simulink model "Contol_PID_OPC_Tanque02"  (R2013a)
settings: Solver=ode45  StartTime=0.0  StopTime=400  RelTol=1e-3
PreLoadFcn:
  | load('Kp.mat')
  | load('Kd.mat')
  | load('Ki.mat')
  | load('Kpm.mat')
  | load('Kdm.mat')
  | load('Kim.mat')
InitFcn:
  | load('Kp.mat')
  | load('Kd.mat')
  | load('Ki.mat')
  | load('Kpm.mat')
  | load('Kdm.mat')
  | load('Kim.mat')
values from neighbouring files (symbols this model uses):
  Kd = -2.1308168557    [Kd.mat]
  Kdm = x(3)    [Funcion_Objetivo_PID.m]    (also in Kdm.mat = 1.60825262821)
  Ki = 0.22046236166    [Kd.mat]
  Kim = x(2)    [Funcion_Objetivo_PID.m]    (also in Kdm.mat = -0.37973848981)
  Kp = 4.86450734815    [Kd.mat]
  Kpm = x(1)    [Funcion_Objetivo_PID.m]    (also in Kdm.mat = 0.790500863568)
undefined symbols (not defined in the file or in its folder): sigbuilder_block
libraries: opclib x4, simulink x2
settings Model: Creator=alvares  LastModifiedBy=alvares

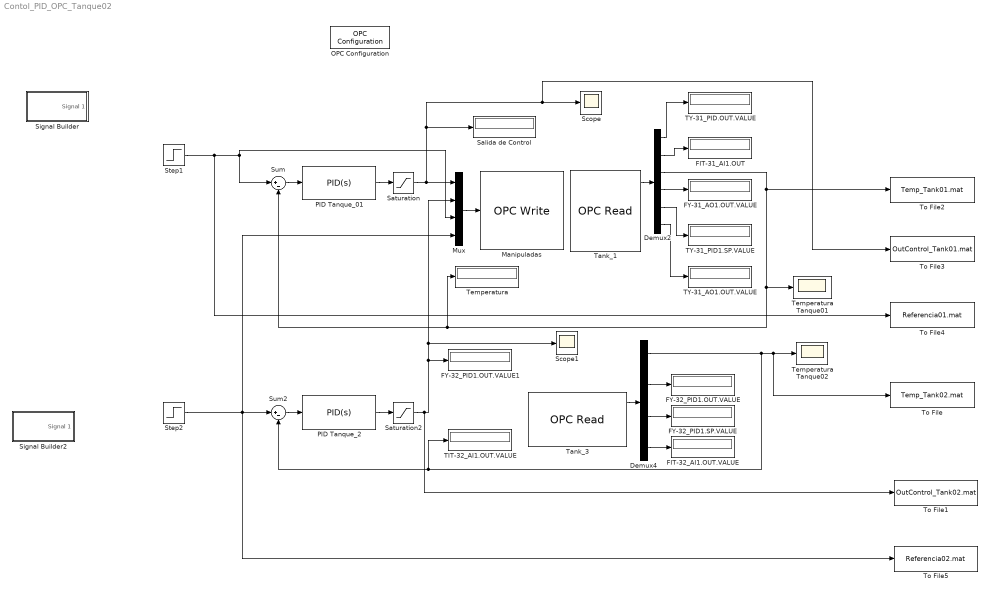
== system Contol_PID_OPC_Tanque02 ==
  Demux2 : Demux  Outputs=6
  Demux4 : Demux
  FIT-31_AI1.OUT : Display
  FIT-32_AI1.OUT.VALUE : Display
  FY-31_AO1.OUT.VALUE : Display
  FY-32_PID1.OUT.VALUE : Display
  FY-32_PID1.OUT.VALUE1 : Display
  FY-32_PID1.SP.VALUE : Display
  Manipuladas : opclib/OPC Write  serverHost=164.41.17.129  serverID=Smar.DfiOleServer.0  itemIDs=TY-31_PID1.OUT.VALUE, FY-32_PID1.OUT.VALUE, TY-31_PID1.SP.VALUE, FY-32_PID1.SP.VALUE  writeMode=Synchronous  updateRate=0.5
  Mux : Mux
  OPC Configuration : opclib/OPC Configuration  opcServers=164.41.17.129/Smar.DfiOleServer.0/10  errMissingItems=Error  errReadWrite=Warn  errShutdown=Error  errRTViolation=Warn  rtEnable=on  speedup=1  showLatency=off  beingUsed=on
  PID Tanque_01 : simulink/Continuous/PID Controller  Controller=PID  TimeDomain=Continuous-time  SampleTime=1  IntegratorMethod=Forward Euler  FilterMethod=Forward Euler  Form=Parallel  P=Kp  I=Ki  D=Kd  N=100  InitialConditionSource=internal  InitialConditionForIntegrator=0  InitialConditionForFilter=0  ExternalReset=none  ZeroCross=off  LimitOutput=off  UpperSaturationLimit=inf  LowerSaturationLimit=-inf  LinearizeAsGain=on  AntiWindupMode=none  Kb=1  TrackingMode=off  Kt=1  PParamMin=[]  PParamMax=[]  IParamMin=[]  IParamMax=[]  DParamMin=[]  DParamMax=[]  NParamMin=[]  NParamMax=[]  KbParamMin=[]  KbParamMax=[]  KtParamMin=[]  KtParamMax=[]  POutMin=[]  POutMax=[]  IOutMin=[]  IOutMax=[]  DOutMin=[]  DOutMax=[]  NOutMin=[]  NOutMax=[]  KbOutMin=[]  KbOutMax=[]  KtOutMin=[]  KtOutMax=[]  IntegratorOutMin=[]  IntegratorOutMax=[]  FilterOutMin=[]  FilterOutMax=[]  SumOutMin=[]  SumOutMax=[]  SumI1OutMin=[]  SumI1OutMax=[]  SumI2OutMin=[]  SumI2OutMax=[]  SumI3OutMin=[]  SumI3OutMax=[]  SumDOutMin=[]  SumDOutMax=[]  SaturationOutMin=[]  SaturationOutMax=[]  IntegratorContinuousStateAttributes=''  IntegratorStateMustResolveToSignalObject=off  IntegratorRTWStateStorageClass=Auto  FilterContinuousStateAttributes=''  FilterStateMustResolveToSignalObject=off  FilterRTWStateStorageClass=Auto
  PID Tanque_2 : simulink/Continuous/PID Controller  Controller=PID  TimeDomain=Continuous-time  SampleTime=1  IntegratorMethod=Forward Euler  FilterMethod=Forward Euler  Form=Parallel  P=Kpm  I=Kim  D=Kdm  N=100  InitialConditionSource=internal  InitialConditionForIntegrator=0  InitialConditionForFilter=0  ExternalReset=none  LimitOutput=off  UpperSaturationLimit=inf  LowerSaturationLimit=-inf  LinearizeAsGain=on  AntiWindupMode=none  Kb=1  TrackingMode=off  Kt=1  PParamMin=[]  PParamMax=[]  IParamMin=[]  IParamMax=[]  DParamMin=[]  DParamMax=[]  NParamMin=[]  NParamMax=[]  KbParamMin=[]  KbParamMax=[]  KtParamMin=[]  KtParamMax=[]  POutMin=[]  POutMax=[]  IOutMin=[]  IOutMax=[]  DOutMin=[]  DOutMax=[]  NOutMin=[]  NOutMax=[]  KbOutMin=[]  KbOutMax=[]  KtOutMin=[]  KtOutMax=[]  IntegratorOutMin=[]  IntegratorOutMax=[]  FilterOutMin=[]  FilterOutMax=[]  SumOutMin=[]  SumOutMax=[]  SumI1OutMin=[]  SumI1OutMax=[]  SumI2OutMin=[]  SumI2OutMax=[]  SumI3OutMin=[]  SumI3OutMax=[]  SumDOutMin=[]  SumDOutMax=[]  SaturationOutMin=[]  SaturationOutMax=[]  IntegratorContinuousStateAttributes=''  IntegratorStateMustResolveToSignalObject=off  IntegratorRTWStateStorageClass=Auto  FilterContinuousStateAttributes=''  FilterStateMustResolveToSignalObject=off  FilterRTWStateStorageClass=Auto
  Salida de Control : Display
  Saturation : Saturate  UpperLimit=100  LowerLimit=-100  ZeroCross=off
  Saturation2 : Saturate  UpperLimit=100  LowerLimit=-100  ZeroCross=off
  Scope : Scope
      settings: SaveName=Saida_PID_AQUECIMENTO
  Scope1 : Scope
      settings: SaveName=Saida_PID_MISTURA
  Signal Builder : Subsystem  Tag=STV Subsys  LoadFcn=sigbuilder_block('load');  StartFcn=sigbuilder_block('start');  StopFcn=sigbuilder_block('stop');  ClipboardFcn=sigbuilder_block('clipboard');  mask(Sigbuilder block){}
      mask help: Simulink:masks:SigbuilderBlock_MD
      mask init:
      | if ~strcmp(get_param(bdroot(gcbh),'SimulationStatus'),'stopped') tuvar = sigbuilder_block('maskInit'); end
      settings: CopyFcn=sigbuilder_block('copy');  DeleteFcn=sigbuilder_block('delete');  ModelCloseFcn=sigbuilder_block('modelClose');  PreSaveFcn=sigbuilder_block('preSave');  PauseFcn=sigbuilder_block('pause');  ContinueFcn=sigbuilder_block('continue');  NameChangeFcn=sigbuilder_block('namechange');  OpenFcn=sigbuilder_block('open',[6 28.5 1012.5 484.5 ]);  CloseFcn=sigbuilder_block('close');
      mask Display: plot(0, 0, 100, 100,[2, 2, 32, 32, 2], [68, 8, 8, 68, 68],[32, 2], [38, 38], [32, 19, 2],[53, 60, 44], [32, 17, 17, 2],[16, 16, 31, 31]);txt = getActiveGroup(gcbh);text(2, 100, txt,'verticalAlignment', 'top');
  Signal Builder2 : Subsystem  Tag=STV Subsys  LoadFcn=sigbuilder_block('load');  StartFcn=sigbuilder_block('start');  StopFcn=sigbuilder_block('stop');  ClipboardFcn=sigbuilder_block('clipboard');  mask(Sigbuilder block){}
      mask help: Simulink:masks:SigbuilderBlock_MD
      mask init:
      | if ~strcmp(get_param(bdroot(gcbh),'SimulationStatus'),'stopped') tuvar = sigbuilder_block('maskInit'); end
      settings: CopyFcn=sigbuilder_block('copy');  DeleteFcn=sigbuilder_block('delete');  ModelCloseFcn=sigbuilder_block('modelClose');  PreSaveFcn=sigbuilder_block('preSave');  PauseFcn=sigbuilder_block('pause');  ContinueFcn=sigbuilder_block('continue');  NameChangeFcn=sigbuilder_block('namechange');  OpenFcn=sigbuilder_block('open',[6 28.5 1012.5 484.5 ]);  CloseFcn=sigbuilder_block('close');
      mask Display: plot(0, 0, 100, 100,[2, 2, 32, 32, 2], [68, 8, 8, 68, 68],[32, 2], [38, 38], [32, 19, 2],[53, 60, 44], [32, 17, 17, 2],[16, 16, 31, 31]);txt = getActiveGroup(gcbh);text(2, 100, txt,'verticalAlignment', 'top');
  Step1 : Step  After=36  SampleTime=0
  Step2 : Step  After=35  SampleTime=0
  Sum : Sum  Inputs=|+-
  Sum2 : Sum  Inputs=|+-
  TIT-32_AI1.OUT.VALUE : Display
  TY-31_AO1.OUT.VALUE : Display
  TY-31_PID.OUT.VALUE : Display
  TY-31_PID1.SP.VALUE : Display
  Tank_1 : opclib/OPC Read  serverHost=164.41.17.129  serverID=Smar.DfiOleServer.0  itemIDs=TY-31_PID1.OUT.VALUE, FIT-31_AI1.OUT, TIT-31_AI1.OUT.VALUE, FY-31_AO1.OUT.VALUE, TY-31_PID1.SP.VALUE, TY-31_AO1.OUT.VALUE  readMode=Synchronous (cache)  dataType=single  updateRate=0.001  showQual=on  showTS=on  tsMode=Seconds since start
  Tank_3 : opclib/OPC Read  serverHost=164.41.17.129  serverID=Smar.DfiOleServer.0  itemIDs=TIT-32_AI1.OUT.VALUE, FY-32_PID1.OUT.VALUE, FY-32_PID1.SP.VALUE, FIT-32_AI1.OUT.VALUE  readMode=Synchronous (cache)  dataType=single  updateRate=0.5  showQual=on  showTS=on  tsMode=Seconds since start
  Temperatura : Display
  Temperatura Tanque01 : Scope
      settings: YMin=36.002  YMax=36.009  SaveName=Tank01_PID_Historial_28
  Temperatura Tanque02 : Scope
      settings: YMin=35.775  YMax=35.81  SaveName=Tank02_PID_History_28
  To File : ToFile  Filename=Temp_Tank02.mat  MatrixName=TempTank02  SaveFormat=Timeseries
  To File1 : ToFile  Filename=OutControl_Tank02.mat  MatrixName=OutPID2  SaveFormat=Timeseries
  To File2 : ToFile  Filename=Temp_Tank01.mat  MatrixName=TempTank01  SaveFormat=Timeseries
  To File3 : ToFile  Filename=OutControl_Tank01.mat  MatrixName=OutPID1  SaveFormat=Timeseries
  To File4 : ToFile  Filename=Referencia01.mat  MatrixName=Refe01  SaveFormat=Timeseries
  To File5 : ToFile  Filename=Referencia02.mat  MatrixName=Refe01  SaveFormat=Timeseries
  wires:
  Mux/1 -> Manipuladas/1
  Demux2/3 -> Sum/2, Temperatura/1, Temperatura Tanque01/1, To File2/1
  Tank_1/1 -> Demux2/1
  Demux4/3 -> FY-32_PID1.SP.VALUE/1
  PID Tanque_01/1 -> Saturation/1
  Sum/1 -> PID Tanque_01/1
  Saturation/1 -> Mux/1, To File3/1, Scope/1, Salida de Control/1
  Demux2/5 -> TY-31_PID1.SP.VALUE/1
  PID Tanque_2/1 -> Saturation2/1
  Saturation2/1 -> To File1/1, FY-32_PID1.OUT.VALUE1/1, Scope1/1, Mux/2
  Sum2/1 -> PID Tanque_2/1
  Tank_3/1 -> Demux4/1
  Demux4/2 -> FY-32_PID1.OUT.VALUE/1
  Demux2/1 -> TY-31_PID.OUT.VALUE/1
  Demux2/2 -> FIT-31_AI1.OUT/1
  Demux2/4 -> FY-31_AO1.OUT.VALUE/1
  Demux2/6 -> TY-31_AO1.OUT.VALUE/1
  Demux4/4 -> FIT-32_AI1.OUT.VALUE/1
  Demux4/1 -> To File/1, Temperatura Tanque02/1, Sum2/2, TIT-32_AI1.OUT.VALUE/1
  Step2/1 -> To File5/1, Mux/4, Sum2/1
  Step1/1 -> To File4/1, Sum/1, Mux/3

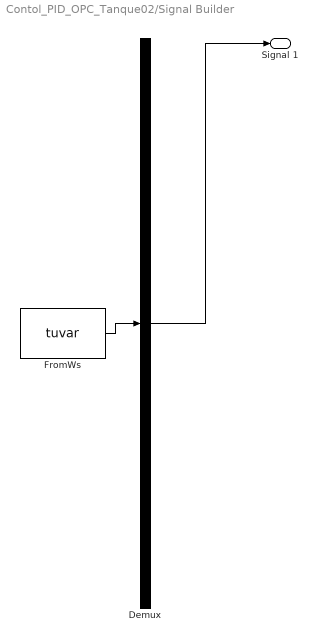
== system Contol_PID_OPC_Tanque02/Signal Builder ==
  Demux : Demux  Tag=STV Demux  Outputs=1
  FromWs : FromWorkspace  Tag=STV FromWs  VariableName=tuvar  SampleTime=0
      SigBuilderData=|
      | common.afterFinalStr = 'Extrapolate'
      | common.sampleTime = 0
      | dataSet.timeRange = [0 300]
      | dataSet.name = 'Group 1'
      | sbobj.Groups.Name = 'Group 1'
      | sbobj.Groups.Signals.Name = 'Signal 1'
      | sbobj.Groups.Signals.XData = [0 200 200 230 275 300]
      | sbobj.Groups.Signals.YData = [42 42 45 45 45 45]
      | sbobj.Groups.TimeRange = [0 300]
  Signal 1 : Outport  Tag=STV Outport
  wires:
  Demux/1 -> Signal 1/1
  FromWs/1 -> Demux/1

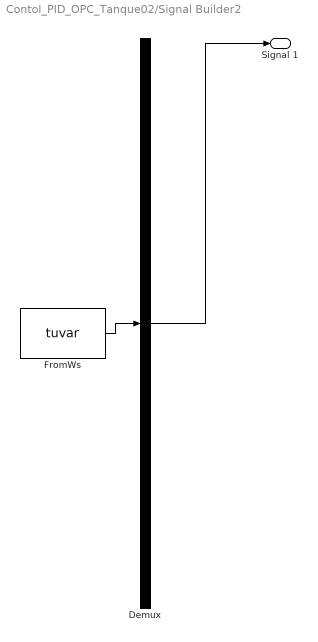
== system Contol_PID_OPC_Tanque02/Signal Builder2 ==
  Demux : Demux  Tag=STV Demux  Outputs=1
  FromWs : FromWorkspace  Tag=STV FromWs  VariableName=tuvar  SampleTime=0
      SigBuilderData=|
      | common.afterFinalStr = 'Extrapolate'
      | common.sampleTime = 0
      | dataSet.timeRange = [0 300]
      | dataSet.name = 'Group 1'
      | sbobj.Groups.Name = 'Group 1'
      | sbobj.Groups.Signals.Name = 'Signal 1'
      | sbobj.Groups.Signals.XData = [0 100 250 250 300]
      | sbobj.Groups.Signals.YData = [38 38 38 34.98 34.98]
      | sbobj.Groups.TimeRange = [0 300]
  Signal 1 : Outport  Tag=STV Outport
  wires:
  Demux/1 -> Signal 1/1
  FromWs/1 -> Demux/1
